simulink model "c221127_FCEV_SLMP_SQP"  (R2022b)
settings: Solver=FixedStepAuto  StartTime=0.0  StopTime=DrvCycLen  FixedStep=1  RelTol=1e-3
values from neighbouring files (symbols this model uses):
  AccThrshd = 1    [Config_c221112.m]    (also in Config_c221127.m; Config_c221218.m; Config_c230117.m; Config_c230321.m)
  AlphaRampFactor = 8    [Config_c221112.m]    (also in Config_c221127.m; Config_c221218.m; Config_c230117.m; Config_c230321.m)
  Bat_eff_chg_average = 0.969    [FCEV_original_data.mat]
  Bat_eff_dis_average = 0.9632    [FCEV_original_data.mat]
  Bat_end_of_life_percent = 20    [FCEV_original_data.mat]
  Bat_I_chg_max = -120    [FCEV_original_data.mat]
  Bat_I_dis_max = 200    [FCEV_original_data.mat]
  Bat_nom_Ic = 2.5    [FCEV_original_data.mat]
  Bat_nom_SOC = 0.35    [FCEV_original_data.mat]
  Bat_nom_temp_oC = 25    [FCEV_original_data.mat]
  Bat_num_pa = 9    [FCEV_original_data.mat]
  Bat_num_se = 97    [FCEV_original_data.mat]
  Bat_ori_C1_chg_F = [397.526659684 455.660832136 435.08783522 460.845064365 457.605812374 417.289828504 416.373906992 359.741413056 321.561704819 1109.14132554 1165.67733205 1135.97600211 ... (72 elements, 9x8)]    [FCEV_original_data.mat]
  Bat_ori_C1_dis_F = [187.121968588 287.083505726 346.448009002 395.529439835 387.517274826 389.973134196 432.856765051 486.92921923 512.158935268 425.990733989 614.68708868 771.472592368 ... (72 elements, 9x8)]    [FCEV_original_data.mat]
  Bat_ori_C2_chg_F = [8748.48589695 7773.35875681 9404.86567646 8934.73981058 8290.58671366 7592.78422269 7759.44623103 7396.59043829 6151.35152293 16187.7227039 11721.8480541 13157.8579836 ... (72 elements, 9x8)]    [FCEV_original_data.mat]
  Bat_ori_C2_dis_F = [2939.81325553 4590.73311898 5504.93546413 5887.5077374 6534.37836712 7765.46899768 10584.7751706 10372.0508438 9238.72693885 5207.86390693 7911.43744944 8879.62137571 ... (72 elements, 9x8)]    [FCEV_original_data.mat]
  Bat_ori_cap_max_Ah = 20.7    [Config_c221218.m]    (also in Config_c230117.m; Config_c230321.m; FCEV_original_data.mat)
  Bat_ori_dUdt4 = [-0.303773584906 -0.249056603774 -0.115094339623 -0.0396226415094 0.0396226415094 0.0641509433962 0.107547169811 0.111320754717 0.0415094339623 0.0547169811321 0.130188679245]    [FCEV_original_data.mat]
  Bat_ori_R0_chg_O = [0.0771669453735 0.0731809311402 0.0726556782939 0.0729965156794 0.0731758310684 0.0742031005051 0.0721266921026 0.0714211058078 0.0714186176143 0.0374124505155 0.0354566732504 0.0345430657188 ... (72 elements, 9x8)]    [FCEV_original_data.mat]
  Bat_ori_R0_dis_O = [0.0819458671157 0.0812429476608 0.0803749674507 0.0805513601722 0.0838629023857 0.0850797840015 0.0829875518672 0.0826388888889 0.0812514106148 0.0428124986417 0.0424658903711 0.0428572670451 ... (72 elements, 9x8)]    [FCEV_original_data.mat]
  Bat_ori_R1_chg_O = [0.114339870884 0.105392753268 0.104421193553 0.109821896183 0.114868279838 0.123333154908 0.129174812826 0.149917249373 0.174896487845 0.0420560161846 0.0390948352938 0.0370122837364 ... (72 elements, 9x8)]    [FCEV_original_data.mat]
  Bat_ori_R1_dis_O = [0.304806399643 0.213604089624 0.171463520004 0.151183840498 0.140630862434 0.128795299077 0.116857791733 0.112567113582 0.106368362501 0.0943235089866 0.0730697254134 0.0611414736086 ... (72 elements, 9x8)]    [FCEV_original_data.mat]
  Bat_ori_R2_chg_O = [0.134518959939 0.17565045702 0.161100627268 0.189032232545 0.205639040497 0.226170473035 0.223651875822 0.181765694192 0.212966950836 0.073628872144 0.0788540822416 0.0792414571734 ... (72 elements, 9x8)]    [FCEV_original_data.mat]
  Bat_ori_R2_dis_O = [0.354968099904 0.285293035102 0.286338708953 0.298763853987 0.248762838155 0.178586175471 0.129047399775 0.188406991173 0.174494800676 0.131839238891 0.123225430215 0.132069033134 ... (72 elements, 9x8)]    [FCEV_original_data.mat]
  Bat_ori_SOC2 = [0 0.001 0.002 0.003 0.004 0.005 0.006 0.007 0.008 0.009 0.01 0.011 ... (1001 elements, 1x1001)]    [FCEV_original_data.mat]
  Bat_ori_SOC4 = [-0.00598301069999 0.0920117618231 0.190864167279 0.289083557951 0.387343788287 0.485011843502 0.5850485992 0.678163031937 0.774810095565 0.876684636119 0.972739524626]    [FCEV_original_data.mat]
  Bat_ori_Uoc_chg_V = [2.4478 2.54923264342 2.6007 2.6383 2.66953057366 2.69636321708 2.7197 2.74042850391 2.75906114733 2.77619379074 2.792 2.80675907757 ... (1001 elements, 1x1001)]    [FCEV_original_data.mat]
  Bat_ori_Uoc_dis_V = [1.9998 2.03916768329 2.24724374236 2.39700902919 2.48767431602 2.5476 2.5882 2.6202 2.64771773167 2.6719 2.6933 2.71251566192 ... (1001 elements, 1x1001)]    [FCEV_original_data.mat]
  Bat_ori_Uoc_V = [2.2238 2.29420016335 2.42397187118 2.5176545146 2.57860244484 2.62198160854 2.65395 2.68031425195 2.7033894395 2.72404689537 2.74265 2.75963736975 ... (1001 elements, 1x1001)]    [FCEV_original_data.mat]
  Bat_power_max_kW = 50    [FCEV_original_data.mat]
  Bat_power_min_kW = 0    [FCEV_original_data.mat]
  Bat_single_capacity_nom_Ah = 2.3    [FCEV_original_data.mat]
  Bat_SOC_ini = 0.3    [Config_c22100601.m]    (also in Config_c22100701.m; FCEV_original_data.mat = 0.45)
  Bat_SOC_max = 0.9    [FCEV_original_data.mat]
  Bat_SOC_min = 0.3    [FCEV_original_data.mat]
  Bat_temp_amb_oC = 25    [FCEV_original_data.mat]
  Bat_temp_cool_oC = 25    [FCEV_original_data.mat]
  BattInitTemp = 25    [Config_c221127.m]    (also in Config_c221218.m; Config_c230117.m; Config_c230321.m)
  BattOnly = 0    [Config_c221218.m]    (also in Config_c230117.m = BattSocRightNow > BattSocLowerLimit; Config_c230321.m = double(BattSocRightNow > BattSocLowerLimit))
  BattSocInit = 0.9    [Config_c221112.m]    (also in Config_c221127.m = 0.3; Config_c221218.m = 0.3; Config_c230117.m = 0.8; Config_c230321.m = 0.8)
  BattSocLowerLimit = 0.25    [Config_c221112.m]    (also in Config_c221127.m = 0.3; Config_c221218.m = 0.3; Config_c230117.m = 0.3; Config_c230321.m = 0.3)
  BattSocRightNow = BattSocRightNow - SocDrop    [Config_c221218.m]    (also in Config_c230117.m; Config_c230321.m)
  BattSocUpperLimit = 0.9    [Config_c221112.m]    (also in Config_c221127.m = 0.8; Config_c221218.m = 0.8; Config_c230117.m = 0.8; Config_c230321.m = 0.8)
  CFWF = 0.5    [Config_c221127.m]    (also in Config_c221218.m; Config_c230117.m; Config_c230321.m)
  DCAC_eff = 0.95    [FCEV_original_data.mat]
  DCDC_ori_eff = [0.95 0.96 0.97 0.976 0.98 0.978 0.973 0.962]    [FCEV_original_data.mat]
  DCDC_ori_power_kW = [0 10 20 30 40 50 60 70]    [FCEV_original_data.mat]
  DeAccThrshd = -1    [Config_c221112.m]    (also in Config_c221127.m; Config_c221218.m; Config_c230117.m; Config_c230321.m)
  DeltaFcPwrRcm_down = 0.5    [Config_c221127.m]    (also in Config_c221218.m; Config_c230117.m; Config_c230321.m)
  DeltaFcPwrRcm_up = 2    [Config_c221127.m]    (also in Config_c221218.m = 3; Config_c230117.m = 4; Config_c230321.m = 4)
  DrvCycRange = sum(DrvCycVps(:,2))    [Config_c221112.m]    (also in Config_c221127.m; Config_c221218.m; Config_c230117.m; Config_c230321.m)
  FC_ori_eff = [0.1 0.33 0.492 0.533 0.559 0.596 0.591 0.562 0.508]    [FCEV_original_data.mat]
  FC_ori_fuel_rate_gps = [0 0.0505050505051 0.0846883468835 0.117260787992 0.149075730471 0.279642058166 0.423011844332 0.593119810202 0.820209973753]    [FCEV_original_data.mat]
  FC_ori_power_kW = [0 2 5 7.5 10 20 30 40 50]    [FCEV_original_data.mat]
  FC_power_max_kW = 50    [FCEV_original_data.mat]
  FC_power_min_kW = 0    [FCEV_original_data.mat]
  FcPwrDropCall = 6    [Config_c221127.m]    (also in Config_c221218.m; Config_c230117.m; Config_c230321.m)
  HydpriceRmb = 30    [Config_c221127.m]    (also in Config_c221218.m; Config_c230117.m; Config_c230321.m)
  m = Time_sample    [Config_c22100601.m]    (also in Config_c22100701.m)
  MC_eff_brk_average = 0.810578512397    [FCEV_original_data.mat]
  MC_eff_dri_average = 0.810578512397    [FCEV_original_data.mat]
  MC_inertia = 0.06    [FCEV_original_data.mat]
  MC_ori_eff = [0.7 0.78 0.85 0.86 0.81 0.82 0.79 0.78 0.78 0.78 0.78 0.7 ... (231 elements, 11x21)]    [FCEV_original_data.mat]
  MC_ori_power_brk_req_kW = [0 -28.3912930389 -56.7825860779 -85.1738791168 -113.565172156 -141.956465195 -170.347758234 -198.739051273 -227.130344311 -255.52163735 -283.912930389 0 ... (121 elements, 11x11)]    [FCEV_original_data.mat]
  MC_ori_power_dri_req_kW = [0 0 0 0 0 0 0 0 0 0 0 0 ... (121 elements, 11x11)]    [FCEV_original_data.mat]
  MC_ori_spd_rpm = [0 1000 2000 3000 4000 5000 6000 7000 8000 9000 10000]    [FCEV_original_data.mat]
  MC_ori_trq_brk_max_Nm = [-271.1368 -271.1368 -271.1368 -237.5159 -178.1369 -142.4824 -118.7579 -101.8119 -89.0685 -79.172 -71.1734]    [FCEV_original_data.mat]
  MC_ori_trq_brk_Nm = [-271.136848522 -244.02316367 -216.909478817 -189.795793965 -162.682109113 -135.568424261 -108.454739409 -81.3410545565 -54.2273697044 -27.1136848522 0]    [FCEV_original_data.mat]
  MC_ori_trq_dri_max_Nm = [271.1368 271.1368 271.1368 237.5159 178.1369 142.4824 118.7579 101.8119 89.0685 79.172 71.1734]    [FCEV_original_data.mat]
  MC_ori_trq_dri_Nm = [0 27.1136848522 54.2273697044 81.3410545565 108.454739409 135.568424261 162.682109113 189.795793965 216.909478817 244.02316367 271.136848522]    [FCEV_original_data.mat]
  MC_ori_trq_Nm = [-271.136848522 -244.02316367 -216.909478817 -189.795793965 -162.682109113 -135.568424261 -108.454739409 -81.3410545565 -54.2273697044 -27.1136848522 0 27.1136848522 ... (21 elements, 1x21)]    [FCEV_original_data.mat]
  MC_power_max_kW = 75    [FCEV_original_data.mat]
  MC_spd_max_rpm = 10000    [FCEV_original_data.mat]
  MC_spd_min_rpm = 0    [FCEV_original_data.mat]
  MC_spd_scale = 1    [FCEV_original_data.mat]
  MC_trq_scale = 1    [FCEV_original_data.mat]
  MC_U_min_V = 120    [FCEV_original_data.mat]
  no_FcPwrSlowDrop = 1    [Config_c230321.m]
  Placeholder = 0    [Config_c221127.m]    (also in Config_c221218.m; Config_c230117.m; Config_c230321.m)
  PredLen = 5    [Config_c221112.m]    (also in Config_c221127.m; Config_c221218.m; Config_c230117.m; Config_c230321.m)
  Road_u = 0.75    [FCEV_original_data.mat]
  SC_np = 1    [Config_c230321.m]
  SC_ns = 100    [Config_c230321.m]
  SC_rc = 1000    [Config_c230321.m]
  SLMP_LearningRate = 0.05    [Config_c221112.m]    (also in Config_c221127.m; Config_c221218.m; Config_c230117.m; Config_c230321.m)
  tDegTable = [zeros(1,3),linspace(0,0.13,47)]    [Config_c221127.m]    (also in Config_c221218.m; Config_c230117.m; Config_c230321.m)
  usd2rmb = 7.116    [Config_c22100601.m]    (also in Config_c22100701.m; Config_c221106.m = 6; Config_c221112.m = 6; Config_c221127.m = 6)
  Veh_air_density_kgpm2 = 1.2    [FCEV_original_data.mat]
  Veh_brk_front = [1 0.6 0.608 0.61 0.618 0.624 0.636 0.645 0.655]    [FCEV_original_data.mat]
  Veh_brk_z = [0.1 0.2 0.3 0.4 0.5 0.6 0.7 0.8 0.9]    [FCEV_original_data.mat]
  Veh_brk_z_max = 0.7    [FCEV_original_data.mat]
  Veh_brk_z_min = 0.1    [FCEV_original_data.mat]
  Veh_coeff_drag = 0.312    [FCEV_original_data.mat]
  Veh_coeff_roll = 0.00863    [FCEV_original_data.mat]
  Veh_final_drive_inertia = 0.1105    [FCEV_original_data.mat]
  Veh_final_drive_ratio = 3.47    [FCEV_original_data.mat]
  Veh_frontal_area_m2 = 2.06    [FCEV_original_data.mat]
  Veh_gravity_acc_ms2 = 9.81    [FCEV_original_data.mat]
  Veh_mass_cargo_kg = 113    [FCEV_original_data.mat]
  Veh_mass_curb_kg = 1157    [FCEV_original_data.mat]
  Veh_mech_eff = 0.9    [FCEV_original_data.mat]
  Veh_rotary_mass_conversion_factor = 1.05    [FCEV_original_data.mat]
  Veh_size_cg_height_m = 0.53    [FCEV_original_data.mat]
  Veh_wheel_inertia = 3.1039    [FCEV_original_data.mat]
  Veh_wheel_radius_m = 0.313    [FCEV_original_data.mat]
  Veh_wt_frac_front = 0.5    [FCEV_original_data.mat]
  VstdThrshd = 2    [Config_c221112.m]    (also in Config_c221127.m; Config_c221218.m; Config_c230117.m; Config_c230321.m)
undefined symbols (not defined in the file or in its folder): Bat_ori_temp, SC_iv, SC_nm, SC_SocTable
libraries: autolibshared x2
(part 3 of 8)

== system c221127_FCEV_SLMP_SQP/VehModel_Current/车轮模型 ==
  "tractive force, brake force and speed req'd of tire/road interface 需求驱动力N 目标车速m/s 需求制动力N" : Inport
  "drive torque (Nm) brake torque (Nm) speed (rad/s) available from drivetrain into axle " : Inport  Port=2
  - : Gain  Gain=Veh_wheel_radius_m
  Add : Sum
  Add1 : Sum
  Add2 : Sum  Inputs=-+
  Add3 : Sum  Inputs=-+
  Constant : Constant  Value=0
  Demux : Demux  Outputs=3
  Demux1 : Demux  Outputs=3
  Gain1 : Gain  Gain=Veh_wheel_radius_m
  Gain2 : Gain  Gain=1/Veh_wheel_radius_m
  Gain3 : Gain  Gain=1/Veh_wheel_radius_m
  Gain4 : Gain  Gain=Veh_wheel_radius_m
  Interia torque : Subsystem
  Interia torque1 : Subsystem
  Mux : Mux  Inputs=3
  Mux3 : Mux  Inputs=3
  Regenerative energy compute : Subsystem
  Saturation : Saturate  UpperLimit=inf  LowerLimit=0
  Saturation1 : Saturate  UpperLimit=0  LowerLimit=-inf
  Scope : Scope
  Switch1 : Switch  Criteria=u2 > Threshold  Threshold=15  SaturateOnIntegerOverflow=off  InputSameDT=off
  Tire slip model : Subsystem
  Tire slip model1 : Subsystem
  axle input speed (rad/s) : Gain  Gain=1/Veh_wheel_radius_m
  drive torque (Nm) speed (rad/s) brake torque (Nm) req'd from drivetrain into axle : Outport  InitialOutput=0
  tractive force (N) brake force (N) linear speed achievable (m/s) : Outport  Port=2  InitialOutput=0
  wires:
  Demux/1 -> Gain1/1
  "tractive force, brake force and speed req'd of tire/road interface 需求驱动力N 目标车速m/s 需求制动力N"/1 -> Demux/1
  "drive torque (Nm) brake torque (Nm) speed (rad/s) available from drivetrain into axle "/1 -> Demux1/1
  Demux1/1 -> Add2/2
  Mux/1 -> drive torque (Nm) speed (rad/s) brake torque (Nm) req'd from drivetrain into axle/1
  Gain1/1 -> Add/2
  Add/1 -> Mux/1
  Add2/1 -> Gain2/1
  Gain2/1 -> Tire slip model/1(In1)
  Mux3/1 -> Scope/1, tractive force (N) brake force (N) linear speed achievable (m/s)/1
  Demux/2 -> axle input speed (rad/s)/1, Interia torque/1(车轮线速度 m/s), Interia torque1/1(车轮线速度 m/s)
  Interia torque/1(inertia torque (Nm)) -> Add2/1, Add/1
  Demux/3 -> Gain4/1
  Gain4/1 -> Add1/1
  Interia torque1/1(inertia torque (Nm)) -> Add3/1, Add1/2
  axle input speed (rad/s)/1 -> Switch1/2, Mux/2
  Switch1/1 -> Mux/3
  Constant/1 -> Switch1/3
  Add1/1 -> Switch1/1
  Saturation/1 -> Mux3/1
  Tire slip model/1(dri_force available in front wheel n) -> Saturation/1
  Tire slip model1/1(brk_force available in front wheel n) -> Saturation1/1
  Saturation1/1 -> Regenerative energy compute/1(motor brk force), Mux3/2
  Gain3/1 -> Tire slip model1/1(In1)
  Demux1/2 -> Add3/2
  Add3/1 -> Gain3/1
  Demux1/3 -> -/1
  -/1 -> Regenerative energy compute/3(spd2), Regenerative energy compute/2(spd), Mux3/3

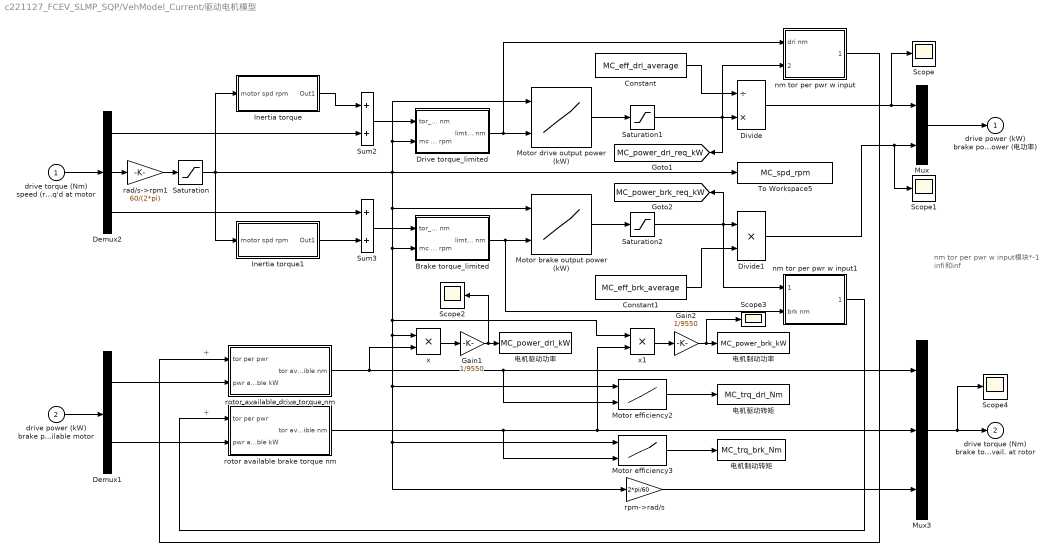
== system c221127_FCEV_SLMP_SQP/VehModel_Current/驱动电机模型 ==
  note: +
  note: +
  note: nm tor per pwr w input模块*-1
      | infi和inf
  drive torque (Nm) speed (rad/s) brake torque (Nm) req'd at motor : Inport
  drive power (kW) brake power (kW) input available motor : Inport  Port=2
  Brake torque_limited : Subsystem
  Constant : Constant  Value=MC_eff_dri_average
  Constant1 : Constant  Value=MC_eff_brk_average
  Demux1 : Demux  Outputs=2
  Demux2 : Demux  Outputs=3
  Divide : Product  Inputs=/*
  Divide1 : Product  Inputs=**
  Drive torque_limited : Subsystem
  Gain1 : Gain  Gain=1/9550
  Gain2 : Gain  Gain=1/9550
  Inertia torque : Subsystem
  Inertia torque1 : Subsystem
  Motor brake output power (kW) : Lookup2D  RowIndex=MC_ori_spd_rpm*MC_spd_scale  ColumnIndex=MC_ori_trq_brk_Nm*MC_trq_scale  Table=MC_ori_power_brk_req_kW*MC_spd_scale*MC_trq_scale
  Motor drive output power (kW) : Lookup2D  RowIndex=MC_ori_spd_rpm*MC_spd_scale  ColumnIndex=MC_ori_trq_dri_Nm*MC_trq_scale  Table=MC_ori_power_dri_req_kW*MC_spd_scale*MC_trq_scale
  Motor efficiency2 : Lookup2D  RowIndex=MC_ori_spd_rpm*MC_spd_scale  ColumnIndex=MC_ori_trq_Nm*MC_trq_scale  Table=MC_ori_eff*MC_spd_scale*MC_trq_scale
  Motor efficiency3 : Lookup2D  RowIndex=MC_ori_spd_rpm*MC_spd_scale  ColumnIndex=MC_ori_trq_Nm*MC_trq_scale  Table=MC_ori_eff*MC_spd_scale*MC_trq_scale
  Mux : Mux  Inputs=2
  Mux3 : Mux  Inputs=3
  Saturation : Saturate  UpperLimit=MC_spd_max_rpm  LowerLimit=MC_spd_min_rpm
  Saturation1 : Saturate  UpperLimit=MC_power_max_kW  LowerLimit=0  LinearizeAsGain=off
  Saturation2 : Saturate  UpperLimit=0  LowerLimit=-MC_power_max_kW
  Scope{,1..4} (5 alike) : Scope
  Sum2 : Sum  InputSameDT=on  SaturateOnIntegerOverflow=on  OutDataTypeStr=Inherit: Same as first input
  Sum3 : Sum  InputSameDT=on  SaturateOnIntegerOverflow=on  OutDataTypeStr=Inherit: Same as first input
  To Workspace5 : ToWorkspace  VariableName=MC_spd_rpm  SampleTime=-1
  nm tor per pwr w input : Subsystem
  nm tor per pwr w input1 : Subsystem
  rad/s->rpm1 : Gain  Gain=60/(2*pi)
  rotor available brake torque nm : Subsystem
  rotor available drive torque nm : Subsystem
  rpm->rad/s : Gain  Gain=2*pi/60
  x : Product  Inputs=**
  x1 : Product  Inputs=**
  电机制动功率 : ToWorkspace  VariableName=MC_power_brk_kW  SampleTime=-1
  电机制动转矩 : ToWorkspace  VariableName=MC_trq_brk_Nm  SampleTime=-1
  电机驱动功率 : ToWorkspace  VariableName=MC_power_dri_kW  SampleTime=-1
  电机驱动转矩 : ToWorkspace  VariableName=MC_trq_dri_Nm  SampleTime=-1
  drive power (kW) brake power (kW) req'd motor input power (电功率) : Outport  InitialOutput=0
  drive torque (Nm) brake torque (Nm) speed avail (rad/s) avail. at rotor : Outport  Port=2  InitialOutput=0
  tag scope: MC_power_brk_req_kW=global, MC_power_dri_req_kW=global
  wires:
  drive torque (Nm) speed (rad/s) brake torque (Nm) req'd at motor/1 -> Demux2/1
  rad/s->rpm1/1 -> Saturation/1
  Demux2/2 -> rad/s->rpm1/1
  Demux2/1 -> Sum2/2
  Inertia torque/1(Out1) -> Sum2/1
  Sum2/1 -> Drive torque_limited/1(tor_req nm)
  Drive torque_limited/1(limted mc torque nm) -> Motor drive output power (kW)/2, nm tor per pwr w input/1(dri nm)
  Motor drive output power (kW)/1 -> Saturation1/1
  Constant/1 -> Divide/1
  Divide/1 -> Scope/1, Mux/1
  Mux/1 -> drive power (kW) brake power (kW) req'd motor input power (电功率)/1
  Demux2/3 -> Sum3/1
  Inertia torque1/1(Out1) -> Sum3/2
  Sum3/1 -> Brake torque_limited/1(tor_req nm)
  Motor brake output power (kW)/1 -> Saturation2/1
  Saturation2/1 -> [MC_power_brk_req_kW], nm tor per pwr w input1/1(pwr brk kW), Divide1/1
  Constant1/1 -> Divide1/2
  Divide1/1 -> Scope1/1, Mux/2
  drive power (kW) brake power (kW) input available motor/1 -> Demux1/1
  Saturation1/1 -> nm tor per pwr w input/2(pwr dri kW), [MC_power_dri_req_kW], Divide/2
  Demux1/1 -> rotor available drive torque nm/2(pwr available kW)
  nm tor per pwr w input/1(tor per pwr) -> rotor available drive torque nm/1(tor per pwr)
  Demux1/2 -> rotor available brake torque nm/2(pwr available kW)
  nm tor per pwr w input1/1(tor per pwr) -> rotor available brake torque nm/1(tor per pwr)
  rotor available brake torque nm/1(tor avaible nm) -> Motor efficiency3/2, x1/2, Mux3/2
  rotor available drive torque nm/1(tor avaible nm) -> Motor efficiency2/2, Mux3/1, x/2
  rpm->rad/s/1 -> Mux3/3
  Motor efficiency3/1 -> 电机制动转矩/1
  Motor efficiency2/1 -> 电机驱动转矩/1
  Brake torque_limited/1(limted mc torque nm) -> nm tor per pwr w input1/2(brk nm), Motor brake output power (kW)/2
  Gain1/1 -> Scope2/1, 电机驱动功率/1
  x/1 -> Gain1/1
  Gain2/1 -> Scope3/1, 电机制动功率/1
  x1/1 -> Gain2/1
  Saturation/1 -> Inertia torque1/1(motor spd rpm), x1/1, x/1, Motor efficiency2/1, Motor efficiency3/1, rpm->rad/s/1, Brake torque_limited/2(mc spd rpm), Motor brake output power (kW)/1, To Workspace5/1, Motor drive output power (kW)/1, Drive torque_limited/2(mc spd rpm), Inertia torque/1(motor spd rpm)
  Mux3/1 -> Scope4/1, drive torque (Nm) brake torque (Nm) speed avail (rad/s) avail. at rotor/1

== system c221127_FCEV_SLMP_SQP/Subsystem2/Capacity Degradation Model (Cell)1/计算实际寿命 ==
  note: 参考文献：A control-oriented cycle-life model for hybrid electric vehicle lithiumion batteries
  note: Beta
  note: Alpha
  温度 : Inport
  倍率 : Inport  Port=2
  SOC : Inport  Port=3
  -31700+163.3*Ic : Sum  InputSameDT=on  SaturateOnIntegerOverflow=on  OutDataTypeStr=Inherit: Same as first input
  Alpha*SOC+Beta1 : Sum  InputSameDT=on  SaturateOnIntegerOverflow=on  OutDataTypeStr=Inherit: Same as first input
  Alpha3 : Constant  Value=2896.6
  Alpha4 : Constant  Value=2649.5
  Beta3 : Constant  Value=7411.2
  Beta4 : Constant  Value=6022.2
  Constant : Constant  Value=-31500
  Constant1 : Constant  Value=152.5
  Constant2 : Constant  Value=273.15
  Fcn2 : Fcn  Expr=u^(1/0.57)
  Math Function : Math  Operator=reciprocal  SignedPower=on
  Math Function1 : Math  Operator=reciprocal  SignedPower=on
  Math Function2 : Math  SignedPower=on
  R : Constant  Value=8.314
  R*T : Product  InputSameDT=on  RndMeth=Zero  SaturateOnIntegerOverflow=on  OutDataTypeStr=Inherit: Same as first input
  Switch3 : Switch  Criteria=u2 > Threshold  Threshold=0.45
  Switch4 : Switch  Criteria=u2 > Threshold  Threshold=0.45
  severity factor function : Product  InputSameDT=on  RndMeth=Zero  SaturateOnIntegerOverflow=on  OutDataTypeStr=Inherit: Same as first input
  x : Product  InputSameDT=on  RndMeth=Zero  SaturateOnIntegerOverflow=on  OutDataTypeStr=Inherit: Same as first input
  x1 : Product  InputSameDT=on  RndMeth=Zero  SaturateOnIntegerOverflow=on  OutDataTypeStr=Inherit: Same as first input
  x2 : Product  InputSameDT=on  RndMeth=Zero  SaturateOnIntegerOverflow=on  OutDataTypeStr=Inherit: Same as first input
  ×1 : Product  InputSameDT=on  RndMeth=Zero  SaturateOnIntegerOverflow=on  OutDataTypeStr=Inherit: Same as first input
  ℃->开氏温度(绝对温度) : Sum  InputSameDT=on  SaturateOnIntegerOverflow=on  OutDataTypeStr=Inherit: Same as first input
  电池标准状态寿命 : ToWorkspace  VariableName=Bat_life_nom  SampleTime=-1
  电池终止寿命(%) : Constant  Value=Bat_end_of_life_percent
  Bat_life_nom : Outport
  wires:
  R/1 -> R*T/1
  ℃->开氏温度(绝对温度)/1 -> R*T/2
  Constant/1 -> -31700+163.3*Ic/1
  x/1 -> -31700+163.3*Ic/2
  Constant1/1 -> x/1
  -31700+163.3*Ic/1 -> x1/1
  R*T/1 -> Math Function/1
  Math Function/1 -> x1/2
  x1/1 -> Math Function2/1
  温度/1 -> ℃->开氏温度(绝对温度)/1
  Constant2/1 -> ℃->开氏温度(绝对温度)/2
  倍率/1 -> x/2
  Math Function2/1 -> severity factor function/1
  Alpha*SOC+Beta1/1 -> severity factor function/2
  severity factor function/1 -> Math Function1/1
  电池终止寿命(%)/1 -> x2/1
  Math Function1/1 -> x2/2
  x2/1 -> Fcn2/1
  Fcn2/1 -> Bat_life_nom/1, 电池标准状态寿命/1
  SOC/1 -> Switch4/2, ×1/1, Switch3/2
  Alpha4/1 -> Switch3/1
  Alpha3/1 -> Switch3/3
  Beta4/1 -> Switch4/1
  Beta3/1 -> Switch4/3
  Switch3/1 -> ×1/2
  Switch4/1 -> Alpha*SOC+Beta1/2
  ×1/1 -> Alpha*SOC+Beta1/1

== system c221127_FCEV_SLMP_SQP/Subsystem2/Capacity Degradation Model (Cell)1/计算电池寿命(标准条件下) ==
  note: 参考文献：A control-oriented cycle-life model for hybrid electric vehicle lithiumion batteries
  note: Beta
  note: Alpha
  标准温度 : Inport
  标准倍率 : Inport  Port=2
  标准SOC : Inport  Port=3
  -31500+152.5*Ic : Sum  InputSameDT=on  SaturateOnIntegerOverflow=on  OutDataTypeStr=Inherit: Same as first input
  Alpha*SOC+Beta : Sum  InputSameDT=on  SaturateOnIntegerOverflow=on  OutDataTypeStr=Inherit: Same as first input
  Alpha3 : Constant  Value=2896.6
  Alpha4 : Constant  Value=2649.5
  Beta3 : Constant  Value=7411.2
  Beta4 : Constant  Value=6022.2
  Constant : Constant  Value=-31500
  Constant1 : Constant  Value=152.5
  Constant2 : Constant  Value=273.15
  Fcn2 : Fcn  Expr=u^(1/0.57)
  Math Function : Math  Operator=reciprocal  SignedPower=on
  Math Function1 : Math  Operator=reciprocal  SignedPower=on
  Math Function2 : Math  SignedPower=on
  R : Constant  Value=8.314
  R*T : Product  InputSameDT=on  RndMeth=Zero  SaturateOnIntegerOverflow=on  OutDataTypeStr=Inherit: Same as first input
  Switch3 : Switch  Criteria=u2 > Threshold  Threshold=0.45
  Switch4 : Switch  Criteria=u2 > Threshold  Threshold=0.45
  severity factor function : Product  InputSameDT=on  RndMeth=Zero  SaturateOnIntegerOverflow=on  OutDataTypeStr=Inherit: Same as first input
  x : Product  InputSameDT=on  RndMeth=Zero  SaturateOnIntegerOverflow=on  OutDataTypeStr=Inherit: Same as first input
  x1 : Product  InputSameDT=on  RndMeth=Zero  SaturateOnIntegerOverflow=on  OutDataTypeStr=Inherit: Same as first input
  x2 : Product  InputSameDT=on  RndMeth=Zero  SaturateOnIntegerOverflow=on  OutDataTypeStr=Inherit: Same as first input
  ×1 : Product  InputSameDT=on  RndMeth=Zero  SaturateOnIntegerOverflow=on  OutDataTypeStr=Inherit: Same as first input
  ℃->开氏温度(绝对温度) : Sum  InputSameDT=on  SaturateOnIntegerOverflow=on  OutDataTypeStr=Inherit: Same as first input
  电池实际状态寿命 : ToWorkspace  VariableName=Bat_life_act  SampleTime=-1
  电池终止寿命(%) : Constant  Value=Bat_end_of_life_percent
  Bat_life_act : Outport
  wires:
  R/1 -> R*T/1
  ℃->开氏温度(绝对温度)/1 -> R*T/2
  Constant/1 -> -31500+152.5*Ic/1
  x/1 -> -31500+152.5*Ic/2
  Constant1/1 -> x/1
  -31500+152.5*Ic/1 -> x1/1
  R*T/1 -> Math Function/1
  Math Function/1 -> x1/2
  x1/1 -> Math Function2/1
  标准温度/1 -> ℃->开氏温度(绝对温度)/1
  Constant2/1 -> ℃->开氏温度(绝对温度)/2
  标准倍率/1 -> x/2
  Math Function2/1 -> severity factor function/1
  Alpha*SOC+Beta/1 -> severity factor function/2
  severity factor function/1 -> Math Function1/1
  电池终止寿命(%)/1 -> x2/1
  Math Function1/1 -> x2/2
  x2/1 -> Fcn2/1
  Fcn2/1 -> Bat_life_act/1, 电池实际状态寿命/1
  标准SOC/1 -> Switch4/2, ×1/1, Switch3/2
  Alpha4/1 -> Switch3/1
  Alpha3/1 -> Switch3/3
  Beta4/1 -> Switch4/1
  Beta3/1 -> Switch4/3
  Switch3/1 -> ×1/2
  Switch4/1 -> Alpha*SOC+Beta/2
  ×1/1 -> Alpha*SOC+Beta/1

== system c221127_FCEV_SLMP_SQP/Subsystem2/Electrical Model1/Current calculation ==
  note: #:电池单体水平
  note: R0chg
  note: R0dis
  Voc : Inport
  Rint : Inport  Port=2
  limited output power (W) : Inport  Port=3
  Constant : Constant  Value=Bat_I_chg_max
  Constant1 : Constant  Value=Bat_I_dis_max
  Constant2 : Constant  Value=0
  Demux : Demux  Outputs=2
  Ibty=(Voc-(Voc^2-4RPbty)^.5) ----------------------------- (2*R) : Fcn  Expr=(u[2]-(u[2]^2-4*u[1]*u[3])^.5)/(2*u[3])
  Ibty=(Voc-(Voc^2-4RPbty)^.5) ----------------------------- (2*R)1 : Fcn  Expr=(u[2]-(u[2]^2-4*u[1]*u[3])^.5)/(2*u[3])
  MinMax : MinMax  Inputs=2
  MinMax1 : MinMax  Function=max  Inputs=2
  Mux : Mux  Inputs=2
  Mux1 : Mux  Inputs=3
  Mux2 : Mux  Inputs=3
  Pbat->Pcell : Gain  Gain=1/(Bat_num_pa*Bat_num_se)  SaturateOnIntegerOverflow=on  OutDataTypeStr=Inherit: Same as input  ParamDataTypeStr=Inherit: Same as input
  Scope : Scope
  Scope1 : Scope
  Switch : Switch  Criteria=u2 > Threshold
  Switch1 : Switch  Criteria=u2 > Threshold  SaturateOnIntegerOverflow=off  InputSameDT=off
  Switch2 : Switch  Criteria=u2 > Threshold
  I_dis (A) I_chg (A) Cell : Outport  InitialOutput=0
  I (A) Cell : Outport  Port=2  InitialOutput=0
  wires:
  Rint/1 -> Demux/1
  limited output power (W)/1 -> Pbat->Pcell/1
  Pbat->Pcell/1 -> Switch/1, Switch/2, Switch2/3, Switch2/2, Switch1/2
  Mux1/1 -> Ibty=(Voc-(Voc^2-4RPbty)^.5) ----------------------------- (2*R)/1
  Demux/1 -> Mux1/3
  Voc/1 -> Mux1/2, Mux2/2
  Demux/2 -> Mux2/3
  Mux2/1 -> Ibty=(Voc-(Voc^2-4RPbty)^.5) ----------------------------- (2*R)1/1
  Ibty=(Voc-(Voc^2-4RPbty)^.5) ----------------------------- (2*R)/1 -> MinMax/2
  Constant1/1 -> MinMax/1
  Ibty=(Voc-(Voc^2-4RPbty)^.5) ----------------------------- (2*R)1/1 -> MinMax1/1
  Constant/1 -> MinMax1/2
  MinMax/1 -> Switch1/1, Mux/1
  MinMax1/1 -> Mux/2, Switch1/3
  Mux/1 -> Scope/1, I_dis (A) I_chg (A) Cell/1
  Switch1/1 -> Scope1/1, I (A) Cell/1
  Switch/1 -> Mux1/1
  Switch2/1 -> Mux2/1
  Constant2/1 -> Switch/3, Switch2/1

== system c221127_FCEV_SLMP_SQP/Subsystem2/Electrical Model1/Entropic Heat ==
  note: 用于计算可逆热
  T : Inport
  SOC : Inport  Port=2
  Constant : Constant  Value=273
  Ent heat : Product  RndMeth=Zero
  Scope : Scope
  Sum2 : Sum  Inputs=|++
  dudT : Lookup  InputValues=Bat_ori_SOC4  Table=Bat_ori_dUdt4  SaturateOnIntegerOverflow=off
  mV->V : Gain  Gain=1/1000
  HG_ent : Outport
  wires:
  Sum2/1 -> Ent heat/2
  Constant/1 -> Sum2/2
  T/1 -> Sum2/1
  dudT/1 -> Ent heat/1
  Ent heat/1 -> mV->V/1
  SOC/1 -> dudT/1
  mV->V/1 -> Scope/1, HG_ent/1

== system c221127_FCEV_SLMP_SQP/Subsystem2/Electrical Model1/Limited power (Battery pack level) ==
  SOC : Inport
  Pbty : Inport  Port=2
  " " : RelationalOperator  Operator=>  OutDataTypeStr=boolean  InputSameDT=off
  " 1" : RelationalOperator  Operator=<  OutDataTypeStr=boolean  InputSameDT=off
  " 3" : Constant  Value=0.95
  Add : Sum
  Constant : Constant  Value=eps
  Constant1 : Constant  Value=eps
  Constant{2..5} (4 alike) : Constant  Value=0
  Logical Operator : Logic  Operator=OR  AllPortsSameDT=off  OutDataTypeStr=boolean
  Logical Operator1 : Logic  AllPortsSameDT=off  OutDataTypeStr=boolean
  Memory1 : Memory  InitialCondition=Bat_SOC_ini  InheritSampleTime=on
  Relational Operator : RelationalOperator  Operator=>  OutDataTypeStr=boolean  InputSameDT=off
  Relational Operator1 : RelationalOperator  OutDataTypeStr=boolean  InputSameDT=off
  Scope : Scope
  Scope1 : Scope  NumInputPorts=2
  Scope2 : Scope  NumInputPorts=2
  Scope3 : Scope
  Switch{,1..3} (4 alike) : Switch  Criteria=u2 > Threshold  Threshold=eps  SaturateOnIntegerOverflow=off  InputSameDT=off
  "Pbty, limited W" : Outport  InitialOutput=0
  wires:
  Memory1/1 -> Relational Operator/1, Relational Operator1/1, Scope3/1
  Constant/1 -> Relational Operator/2
  Relational Operator/1 -> Logical Operator/1
  Switch3/1 -> Scope2/2, " 1"/1, Switch1/3
  Constant1/1 -> " "/2
  " "/1 -> Logical Operator/2
  Logical Operator/1 -> Switch/2
  Constant2/1 -> Switch/3
  " 3"/1 -> Relational Operator1/2
  Relational Operator1/1 -> Logical Operator1/1
  Logical Operator1/1 -> Switch1/2
  Constant3/1 -> Switch1/1
  Constant4/1 -> " 1"/2
  " 1"/1 -> Logical Operator1/2
  Switch2/1 -> Scope2/1, " "/1, Switch/1
  Add/1 -> Scope/1, "Pbty, limited W"/1
  Switch/1 -> Scope1/1, Add/1
  Switch1/1 -> Add/2, Scope1/2
  Pbty/1 -> Switch2/1, Switch3/3, Switch3/2, Switch2/2
  Constant5/1 -> Switch3/1, Switch2/3
  SOC/1 -> Memory1/1

== system c221127_FCEV_SLMP_SQP/Subsystem2/Electrical Model1/Max power in W (Battery pack level) ==
  Constant3 : Constant  Value=Bat_I_dis_max
  Constant4 : Constant  Value=Bat_I_chg_max
  Max power in W (Battery pack level)1 : Subsystem
  Mux1 : Mux  Inputs=3
  Mux2 : Mux  Inputs=3
  Product : Product  InputSameDT=on  RndMeth=Zero  SaturateOnIntegerOverflow=on  OutDataTypeStr=Inherit: Same as first input
  Product1 : Product  InputSameDT=on  RndMeth=Zero  SaturateOnIntegerOverflow=on  OutDataTypeStr=Inherit: Same as first input
  R0,cell->R0,bat : Gain  Gain=Bat_num_se/Bat_num_pa  SaturateOnIntegerOverflow=on  OutDataTypeStr=Inherit: Same as input  ParamDataTypeStr=Inherit: Same as input
  R0,cell->R0,bat1 : Gain  Gain=Bat_num_se/Bat_num_pa  SaturateOnIntegerOverflow=on  OutDataTypeStr=Inherit: Same as input  ParamDataTypeStr=Inherit: Same as input
  fun : Fcn  Expr=u[2]-u[1]*u[3]
  fun1 : Fcn  Expr=u[2]-u[1]*u[3]
  max ess discharge pwr : Outport  InitialOutput=0
  max ess charge pwr : Outport  Port=2  InitialOutput=0
  wires:
  [Bat_R0_dis_O] -> R0,cell->R0,bat/1
  [Bat_R0_chg_O] -> R0,cell->R0,bat1/1
  Constant4/1 -> Product1/1, Mux2/1
  Constant3/1 -> Product/1, Mux1/1
  R0,cell->R0,bat/1 -> Mux1/3
  [Bat_Uoc_V] -> Mux2/2, Mux1/2
  Mux1/1 -> fun/1
  R0,cell->R0,bat1/1 -> Mux2/3
  Mux2/1 -> fun1/1
  fun/1 -> Product/2
  Product/1 -> max ess discharge pwr/1
  fun1/1 -> Product1/2
  Product1/1 -> max ess charge pwr/1

== system c221127_FCEV_SLMP_SQP/Subsystem2/Electrical Model1/Parameter Lookup2 ==
  note: #Cell Level
  SOC : Inport
  T : Inport  Port=2
  P : Inport  Port=3
  Gain{1..5} (5 alike) : Gain
  Lookup C1 : Subsystem
  Lookup C2 : Subsystem
  Lookup R1 : Subsystem
  Lookup R2 : Subsystem
  Lookup Rs : Subsystem
  Lookup Uoc : Subsystem
  Uoc : Outport
  R1 : Outport  Port=2
  C1 : Outport  Port=3
  R2 : Outport  Port=4
  C2 : Outport  Port=5
  R0 : Outport  Port=6
  wires:
  [BattSoc] -> Lookup Rs/1(SOC), Lookup R1/1(SOC), Lookup C1/1(SOC), Lookup Uoc/1(SOC), Lookup C2/1(SOC), Lookup R2/1(SOC1)
  [BattTemp] -> Lookup Rs/2(T), Lookup R1/2(T), Lookup C1/2(T), Lookup C2/2(T), Lookup R2/2(T)
  [BattPwr] -> Lookup R1/3(P), Lookup C1/3(P), Lookup C2/3(P), Lookup Uoc/2(P), Lookup R2/3(P)
  Gain3/1 -> C1/1
  Lookup C2/1(C2) -> Gain4/1
  Gain4/1 -> C2/1
  Gain2/1 -> R2/1
  Lookup R2/1(R2) -> Gain2/1
  Gain1/1 -> R1/1
  Lookup R1/1(R1) -> Gain1/1
  Lookup C1/1(C1) -> Gain3/1
  Lookup Uoc/1(Uoc) -> Gain5/1
  Gain5/1 -> Uoc/1
  Lookup Rs/1(R0) -> R0/1
  SOC/1 -> [BattSoc]
  T/1 -> [BattTemp]
  P/1 -> [BattPwr]

== system c221127_FCEV_SLMP_SQP/Subsystem2/Electrical Model1/SOC Calculation ==
  note: 充电
  note: 放电
  note: #:电池组水平
  I_dis (A) I_chg (A) : Inport
  (sec->hrs) : Gain  Gain=1/3600  SaturateOnIntegerOverflow=on  OutDataTypeStr=Inherit: Same as input  ParamDataTypeStr=Inherit: Same as input
  0 <= SOC <= 1 : Saturate  UpperLimit=1  LowerLimit=eps
  Add5 : Sum  Inputs=-+
  Add6 : Sum  Inputs=-+
  Bat SOC0 : Constant  Value=BattSocInit
  Bat chg eff : Constant  Value=Bat_eff_chg_average
  Bat dis eff : Constant  Value=Bat_eff_dis_average
  CD/CS mode judgement : Subsystem
  Demux : Demux  Outputs=2
  Divide1 : Product  Inputs=*/
  Divide3 : Product  Inputs=**
  Divide4 : Product  Inputs=*/
  Icell->Ibat : Gain  Gain=Bat_num_pa  SaturateOnIntegerOverflow=on  OutDataTypeStr=Inherit: Same as input  ParamDataTypeStr=Inherit: Same as input
  Icell->Ibat1 : Gain  Gain=Bat_num_pa  SaturateOnIntegerOverflow=on  OutDataTypeStr=Inherit: Same as input  ParamDataTypeStr=Inherit: Same as input
  Integrator1 : Integrator  InitialCondition=eps
  Integrator6 : Integrator
  Integrator7 : Integrator
  Product3 : Product  RndMeth=Zero
  Product4 : Product  RndMeth=Zero
  Q0 : Constant  Value=Bat_ori_cap_max_Ah
  Scope : Scope
  Switch : Switch  Criteria=u2 > Threshold  SaturateOnIntegerOverflow=off  InputSameDT=off
  To Workspace3 : ToWorkspace  VariableName=Energy_bat_consume_kWh  SaveFormat=Timeseries  SampleTime=-1
  Ws->kWh : Gain  Gain=-1/(1000*3600)
  Ws->kWh1 : Gain  Gain=-1/(1000*3600)
  SOC : Outport  InitialOutput=0
  wires:
  0 <= SOC <= 1/1 -> CD/CS mode judgement/1(SOC), SOC/1
  I_dis (A) I_chg (A)/1 -> Scope/1, Demux/1
  Demux/1 -> Icell->Ibat/1
  Demux/2 -> Icell->Ibat1/1
  Divide3/1 -> Switch/2, Product3/1, Switch/1
  Icell->Ibat/1 -> Divide3/1
  Bat dis eff/1 -> Divide3/2
  Bat chg eff/1 -> Divide4/2
  Icell->Ibat1/1 -> Divide4/1
  Divide4/1 -> Product4/2, Switch/3
  Add5/1 -> 0 <= SOC <= 1/1
  [Bat_Uoc_V] -> Product4/1, Product3/2
  Add6/1 -> To Workspace3/1
  Product3/1 -> Integrator6/1
  Integrator6/1 -> Ws->kWh/1
  Ws->kWh/1 -> Add6/1
  Product4/1 -> Integrator7/1
  Integrator7/1 -> Ws->kWh1/1
  Ws->kWh1/1 -> Add6/2
  Switch/1 -> (sec->hrs)/1
  (sec->hrs)/1 -> Integrator1/1
  Integrator1/1 -> Divide1/1
  Q0/1 -> Divide1/2
  Bat SOC0/1 -> Add5/2
  Divide1/1 -> Add5/1

== system c221127_FCEV_SLMP_SQP/Subsystem2/Electrical Model1/U0 ==
  R0 : Inport
  I : Inport  Port=2
  Demux : Demux  Outputs=2
  Switch : Switch  Criteria=u2 > Threshold  SaturateOnIntegerOverflow=off  InputSameDT=off
  U0=I*R0 : Product  RndMeth=Zero
  U0 : Outport
  wires:
  I/1 -> U0=I*R0/2, Switch/2
  R0/1 -> Demux/1
  Demux/1 -> Switch/1
  Demux/2 -> Switch/3
  Switch/1 -> U0=I*R0/1
  U0=I*R0/1 -> U0/1

== system c221127_FCEV_SLMP_SQP/Subsystem2/Electrical Model1/U1&U1 ==
  note: -V2/(C2*R2)+I/C2
  note: -V1/(C1*R1)+I/C1
  R1 : Inport
  C1 : Inport  Port=2
  R2 : Inport  Port=3
  C2 : Inport  Port=4
  I : Inport  Port=5
  Delay : Delay  DelayLength=1
  Ib/C1 : Product  Inputs=*/  RndMeth=Zero
  Ib/C2 : Product  Inputs=*/  RndMeth=Zero
  Memory1 : Memory  InitialCondition=eps  InheritSampleTime=on
  R1*C1 : Product  Inputs=**  RndMeth=Zero
  R2*C2 : Product  Inputs=**  RndMeth=Zero
  Scope : Scope  NumInputPorts=2
  Scope1 : Scope
  Sum1 : Sum
  Sum2 : Sum  Inputs=|-+
  Sum3 : Sum  Inputs=+-|
  Sum4 : Sum
  U1/(R1*C1) : Product  Inputs=*/  RndMeth=Zero
  U2/(R2*C2) : Product  Inputs=*/  RndMeth=Zero
  U1 : Outport
  U2 : Outport  Port=2
  wires:
  C1/1 -> R1*C1/1, Ib/C1/2
  I/1 -> Scope1/1, Ib/C2/1, Ib/C1/1
  R1/1 -> R1*C1/2
  R1*C1/1 -> U1/(R1*C1)/2
  U1/(R1*C1)/1 -> Sum3/2
  Ib/C1/1 -> Sum3/1
  R2/1 -> R2*C2/1
  C2/1 -> Ib/C2/2, R2*C2/2
  R2*C2/1 -> U2/(R2*C2)/2
  Ib/C2/1 -> Sum2/2
  U2/(R2*C2)/1 -> Sum2/1
  Memory1/1 -> Sum4/1, U2/(R2*C2)/1
  Sum3/1 -> Sum1/1
  Sum1/1 -> Delay/1, Scope/1, U1/1
  Sum2/1 -> Sum4/2
  Sum4/1 -> Scope/2, Memory1/1, U2/1
  Delay/1 -> U1/(R1*C1)/1, Sum1/2

== system c221127_FCEV_SLMP_SQP/Subsystem2/Thermal Model1/Calculation ==
  Cc1 : Constant  Value=62.7
  Cs : Constant  Value=4.5
  "Rc " : Constant  Value=1.94
  Rc*Cc : Product  Inputs=**  RndMeth=Zero
  Rc*Cs : Product  Inputs=**  RndMeth=Zero
  Rs : Constant  Value=3.19
  Rs*Cs : Product  Inputs=**  RndMeth=Zero
  Cc : Outport
  RcCc : Outport  Port=2
  RsCs : Outport  Port=3
  RcCs : Outport  Port=4
  wires:
  Cc1/1 -> Cc/1, Rc*Cc/1
  "Rc "/1 -> Rc*Cc/2, Rc*Cs/1
  Rc*Cc/1 -> RcCc/1
  Cs/1 -> Rs*Cs/1, Rc*Cs/2
  Rs/1 -> Rs*Cs/2
  Rc*Cs/1 -> RcCs/1
  Rs*Cs/1 -> RsCs/1

== system c221127_FCEV_SLMP_SQP/Subsystem3/FcDegCountingSubSys/Subsystem ==
  Enable : EnablePort
  Add : Sum
  Constant : Constant
  Memory : Memory
  u : Outport
  wires:
  Constant/1 -> Add/1
  Add/1 -> Memory/1
  Memory/1 -> Add/2, u/1

== system c221127_FCEV_SLMP_SQP/Subsystem3/FcDegCountingSubSys/Subsystem1 ==
  Enable : EnablePort
  Add : Sum
  Constant : Constant
  Memory : Memory
  u : Outport
  wires:
  Memory/1 -> u/1, Add/2
  Add/1 -> Memory/1
  Constant/1 -> Add/1

== system c221127_FCEV_SLMP_SQP/Subsystem4/VehModel_Pred+1/Power bus ==
  note: -
  note: +
  note: 需求制动功率
  note: 需求驱动功率
  drive power (kW) brake power (kW) req at power bus : Inport
  Constant1 : Constant  Value=DCAC_eff
  Demux2 : Demux  Outputs=2
  Divide : Product  Inputs=*/
  Divide1 : Product  Inputs=**
  Saturation : Saturate  UpperLimit=0  LowerLimit=-inf
  Saturation1 : Saturate  UpperLimit=inf  LowerLimit=0
  Switch1 : Switch  Criteria=u2 > Threshold  SaturateOnIntegerOverflow=off  InputSameDT=off
  drive power (kW)/brake power (kW) req from power sources : Outport
  wires:
  Constant1/1 -> Divide1/2, Divide/2
  Divide/1 -> Saturation1/1
  Divide1/1 -> Saturation/1
  drive power (kW) brake power (kW) req at power bus/1 -> Demux2/1
  Demux2/2 -> Divide1/1
  Saturation1/1 -> Switch1/2, Switch1/1
  Switch1/1 -> drive power (kW)/brake power (kW) req from power sources/1
  Saturation/1 -> Switch1/3
  Demux2/1 -> Divide/1

== system c221127_FCEV_SLMP_SQP/Subsystem4/VehModel_Pred+1/主减及变速器模型 ==
  drive torque (Nm) speed (rad/s) brake torque (Nm) req'd at output side of final drive : Inport
  " Effect of inertia (Nm)1" : Subsystem
  Demux4 : Demux  Outputs=3
  Effect of inertia (Nm) : Subsystem
  Gain1 : Gain  Gain=1/Veh_final_drive_ratio
  Gain2 : Gain  Gain=1/Veh_final_drive_ratio
  Gain3 : Gain  Gain=Veh_final_drive_ratio  SaturateOnIntegerOverflow=on  OutDataTypeStr=Inherit: Same as input  ParamDataTypeStr=Inherit: Same as input
  Mux4 : Mux  Inputs=3
  Sum : Sum  Inputs=+++  InputSameDT=on  SaturateOnIntegerOverflow=on  OutDataTypeStr=Inherit: Same as first input
  Sum3 : Sum  Inputs=+++  InputSameDT=on  SaturateOnIntegerOverflow=on  OutDataTypeStr=Inherit: Same as first input
  loss (Nm) : Subsystem
  loss (Nm)1 : Subsystem
  drive torque (Nm) speed (rad/s) brike torque (Nm) req'd at input side of final drive : Outport  InitialOutput=0
  wires:
  Demux4/2 -> Effect of inertia (Nm)/1(fd input speed (rad/s)), " Effect of inertia (Nm)1"/1(In1), Gain3/1
  Demux4/1 -> loss (Nm)/1("drive torque (Nm) "), Gain1/1
  Mux4/1 -> drive torque (Nm) speed (rad/s) brike torque (Nm) req'd at input side of final drive/1
  drive torque (Nm) speed (rad/s) brake torque (Nm) req'd at output side of final drive/1 -> Demux4/1
  Effect of inertia (Nm)/1(drag torque (Nm)) -> Sum/2
  loss (Nm)/1(drag torque (Nm)) -> Sum/1
  Gain1/1 -> Sum/3
  Sum/1 -> Mux4/1
  Gain3/1 -> Mux4/2
  " Effect of inertia (Nm)1"/1(Out1) -> Sum3/2
  loss (Nm)1/1(drag torque (Nm)) -> Sum3/3
  Demux4/3 -> Gain2/1, loss (Nm)1/1("drive torque (Nm) ")
  Gain2/1 -> Sum3/1
  Sum3/1 -> Mux4/3

== system c221127_FCEV_SLMP_SQP/Subsystem4/VehModel_Pred+1/整车动力学模型 ==
  需求车速 km/h : Inport
  Add1 : Sum  Inputs=++++
  Mux : Mux  Inputs=3
  compute of front axle brk from motor : Subsystem
  kmph->m/s : Gain  Gain=1/3.6
  加速阻力 : Subsystem
  坡度 : Constant  Value=0
  坡道阻力 : Subsystem
  平均车速 km/h : Scope
  整车需求驱动力 : Scope
  滚动阻力 : Subsystem
  空气阻力 : Subsystem
  需求驱动力N 目标车速m/s 需求制动力N : Outport
  wires:
  滚动阻力/1(滚动阻力 N) -> Add1/1
  坡道阻力/1(坡道阻力 N) -> Add1/2
  空气阻力/1(空气阻力 N) -> Add1/3
  加速阻力/1(加速阻力 N) -> Add1/4
  Add1/1 -> 整车需求驱动力/1, Mux/1
  Mux/1 -> 需求驱动力N 目标车速m/s 需求制动力N/1
  坡度/1 -> 坡道阻力/2(预测坡度), 滚动阻力/2(预测坡度)
  kmph->m/s/1 -> Mux/2
  需求车速 km/h/1 -> compute of front axle brk from motor/1(平均车速 km/h), kmph->m/s/1, 平均车速 km/h/1, 加速阻力/1(车速 km/h), 空气阻力/1(veh_spd km/h), 滚动阻力/1(车辆平均车速 km/h), 坡道阻力/1(车辆平均车速1)
  compute of front axle brk from motor/1(veh_front_axle_motor_brk) -> Mux/3

== system c221127_FCEV_SLMP_SQP/Subsystem4/VehModel_Pred+1/车轮模型 ==
  "tractive force, brake force and speed req'd of tire/road interface 需求驱动力N 目标车速m/s 需求制动力N" : Inport
  Add : Sum
  Add1 : Sum
  Constant : Constant  Value=0
  Demux : Demux  Outputs=3
  Gain1 : Gain  Gain=Veh_wheel_radius_m
  Gain4 : Gain  Gain=Veh_wheel_radius_m
  Interia torque : Subsystem
  Interia torque1 : Subsystem
  Mux : Mux  Inputs=3
  Switch1 : Switch  Criteria=u2 > Threshold  Threshold=15  SaturateOnIntegerOverflow=off  InputSameDT=off
  axle input speed (rad/s) : Gain  Gain=1/Veh_wheel_radius_m
  drive torque (Nm) speed (rad/s) brake torque (Nm) req'd from drivetrain into axle : Outport  InitialOutput=0
  wires:
  Demux/1 -> Gain1/1
  "tractive force, brake force and speed req'd of tire/road interface 需求驱动力N 目标车速m/s 需求制动力N"/1 -> Demux/1
  Mux/1 -> drive torque (Nm) speed (rad/s) brake torque (Nm) req'd from drivetrain into axle/1
  Gain1/1 -> Add/2
  Add/1 -> Mux/1
  Demux/2 -> axle input speed (rad/s)/1, Interia torque/1(车轮线速度 m/s), Interia torque1/1(车轮线速度 m/s)
  Interia torque/1(inertia torque (Nm)) -> Add/1
  Demux/3 -> Gain4/1
  Gain4/1 -> Add1/1
  Interia torque1/1(inertia torque (Nm)) -> Add1/2
  axle input speed (rad/s)/1 -> Switch1/2, Mux/2
  Switch1/1 -> Mux/3
  Constant/1 -> Switch1/3
  Add1/1 -> Switch1/1

== system c221127_FCEV_SLMP_SQP/Subsystem4/VehModel_Pred+1/驱动电机模型 ==
  note: nm tor per pwr w input模块*-1
      | infi和inf
  drive torque (Nm) speed (rad/s) brake torque (Nm) req'd at motor : Inport
  Brake torque_limited : Subsystem
  Constant : Constant  Value=MC_eff_dri_average
  Constant1 : Constant  Value=MC_eff_brk_average
  Demux2 : Demux  Outputs=3
  Divide : Product  Inputs=/*
  Divide1 : Product  Inputs=**
  Drive torque_limited : Subsystem
  Inertia torque : Subsystem
  Inertia torque1 : Subsystem
  Motor brake output power (kW) : Lookup2D  RowIndex=MC_ori_spd_rpm*MC_spd_scale  ColumnIndex=MC_ori_trq_brk_Nm*MC_trq_scale  Table=MC_ori_power_brk_req_kW*MC_spd_scale*MC_trq_scale
  Motor drive output power (kW) : Lookup2D  RowIndex=MC_ori_spd_rpm*MC_spd_scale  ColumnIndex=MC_ori_trq_dri_Nm*MC_trq_scale  Table=MC_ori_power_dri_req_kW*MC_spd_scale*MC_trq_scale
  Mux : Mux  Inputs=2
  Saturation : Saturate  UpperLimit=MC_spd_max_rpm  LowerLimit=MC_spd_min_rpm
  Saturation1 : Saturate  UpperLimit=MC_power_max_kW  LowerLimit=0  LinearizeAsGain=off
  Saturation2 : Saturate  UpperLimit=0  LowerLimit=-MC_power_max_kW
  Sum2 : Sum  InputSameDT=on  SaturateOnIntegerOverflow=on  OutDataTypeStr=Inherit: Same as first input
  Sum3 : Sum  InputSameDT=on  SaturateOnIntegerOverflow=on  OutDataTypeStr=Inherit: Same as first input
  rad/s->rpm1 : Gain  Gain=60/(2*pi)
  drive power (kW) brake power (kW) req'd motor input power (电功率) : Outport  InitialOutput=0
  wires:
  drive torque (Nm) speed (rad/s) brake torque (Nm) req'd at motor/1 -> Demux2/1
  rad/s->rpm1/1 -> Saturation/1
  Demux2/2 -> rad/s->rpm1/1
  Demux2/1 -> Sum2/2
  Inertia torque/1(Out1) -> Sum2/1
  Sum2/1 -> Drive torque_limited/1(tor_req nm)
  Drive torque_limited/1(limted mc torque nm) -> Motor drive output power (kW)/2
  Motor drive output power (kW)/1 -> Saturation1/1
  Constant/1 -> Divide/1
  Divide/1 -> Mux/1
  Mux/1 -> drive power (kW) brake power (kW) req'd motor input power (电功率)/1
  Demux2/3 -> Sum3/1
  Inertia torque1/1(Out1) -> Sum3/2
  Sum3/1 -> Brake torque_limited/1(tor_req nm)
  Motor brake output power (kW)/1 -> Saturation2/1
  Saturation2/1 -> Divide1/1
  Constant1/1 -> Divide1/2
  Divide1/1 -> Mux/2
  Saturation1/1 -> Divide/2
  Brake torque_limited/1(limted mc torque nm) -> Motor brake output power (kW)/2
  Saturation/1 -> Inertia torque1/1(motor spd rpm), Brake torque_limited/2(mc spd rpm), Motor brake output power (kW)/1, Motor drive output power (kW)/1, Drive torque_limited/2(mc spd rpm), Inertia torque/1(motor spd rpm)

== system c221127_FCEV_SLMP_SQP/Subsystem4/VehModel_Pred+2/Power bus ==
  note: -
  note: +
  note: 需求制动功率
  note: 需求驱动功率
  drive power (kW) brake power (kW) req at power bus : Inport
  Constant1 : Constant  Value=DCAC_eff
  Demux2 : Demux  Outputs=2
  Divide : Product  Inputs=*/
  Divide1 : Product  Inputs=**
  Saturation : Saturate  UpperLimit=0  LowerLimit=-inf
  Saturation1 : Saturate  UpperLimit=inf  LowerLimit=0
  Switch1 : Switch  Criteria=u2 > Threshold  SaturateOnIntegerOverflow=off  InputSameDT=off
  drive power (kW)/brake power (kW) req from power sources : Outport
  wires:
  Constant1/1 -> Divide1/2, Divide/2
  Divide/1 -> Saturation1/1
  Divide1/1 -> Saturation/1
  drive power (kW) brake power (kW) req at power bus/1 -> Demux2/1
  Demux2/2 -> Divide1/1
  Saturation1/1 -> Switch1/2, Switch1/1
  Switch1/1 -> drive power (kW)/brake power (kW) req from power sources/1
  Saturation/1 -> Switch1/3
  Demux2/1 -> Divide/1

== system c221127_FCEV_SLMP_SQP/Subsystem4/VehModel_Pred+2/主减及变速器模型 ==
  drive torque (Nm) speed (rad/s) brake torque (Nm) req'd at output side of final drive : Inport
  " Effect of inertia (Nm)1" : Subsystem
  Demux4 : Demux  Outputs=3
  Effect of inertia (Nm) : Subsystem
  Gain1 : Gain  Gain=1/Veh_final_drive_ratio
  Gain2 : Gain  Gain=1/Veh_final_drive_ratio
  Gain3 : Gain  Gain=Veh_final_drive_ratio  SaturateOnIntegerOverflow=on  OutDataTypeStr=Inherit: Same as input  ParamDataTypeStr=Inherit: Same as input
  Mux4 : Mux  Inputs=3
  Sum : Sum  Inputs=+++  InputSameDT=on  SaturateOnIntegerOverflow=on  OutDataTypeStr=Inherit: Same as first input
  Sum3 : Sum  Inputs=+++  InputSameDT=on  SaturateOnIntegerOverflow=on  OutDataTypeStr=Inherit: Same as first input
  loss (Nm) : Subsystem
  loss (Nm)1 : Subsystem
  drive torque (Nm) speed (rad/s) brike torque (Nm) req'd at input side of final drive : Outport  InitialOutput=0
  wires:
  Demux4/2 -> Effect of inertia (Nm)/1(fd input speed (rad/s)), " Effect of inertia (Nm)1"/1(In1), Gain3/1
  Demux4/1 -> loss (Nm)/1("drive torque (Nm) "), Gain1/1
  Mux4/1 -> drive torque (Nm) speed (rad/s) brike torque (Nm) req'd at input side of final drive/1
  drive torque (Nm) speed (rad/s) brake torque (Nm) req'd at output side of final drive/1 -> Demux4/1
  Effect of inertia (Nm)/1(drag torque (Nm)) -> Sum/2
  loss (Nm)/1(drag torque (Nm)) -> Sum/1
  Gain1/1 -> Sum/3
  Sum/1 -> Mux4/1
  Gain3/1 -> Mux4/2
  " Effect of inertia (Nm)1"/1(Out1) -> Sum3/2
  loss (Nm)1/1(drag torque (Nm)) -> Sum3/3
  Demux4/3 -> Gain2/1, loss (Nm)1/1("drive torque (Nm) ")
  Gain2/1 -> Sum3/1
  Sum3/1 -> Mux4/3

== system c221127_FCEV_SLMP_SQP/Subsystem4/VehModel_Pred+2/整车动力学模型 ==
  需求车速 km/h : Inport
  Temp : Inport  Port=2
  Add1 : Sum  Inputs=++++
  Mux : Mux  Inputs=3
  compute of front axle brk from motor : Subsystem
  kmph->m/s : Gain  Gain=1/3.6
  加速阻力 : Subsystem
  坡度 : Constant  Value=0
  坡道阻力 : Subsystem
  平均车速 km/h : Scope
  整车需求驱动力 : Scope
  滚动阻力 : Subsystem
  空气阻力 : Subsystem
  需求驱动力N 目标车速m/s 需求制动力N : Outport
  wires:
  滚动阻力/1(滚动阻力 N) -> Add1/1
  坡道阻力/1(坡道阻力 N) -> Add1/2
  空气阻力/1(空气阻力 N) -> Add1/3
  需求车速 km/h/1 -> compute of front axle brk from motor/1(平均车速 km/h), kmph->m/s/1, 平均车速 km/h/1, 加速阻力/1(车速 km/h), 空气阻力/1(veh_spd km/h), 滚动阻力/1(车辆平均车速 km/h), 坡道阻力/1(车辆平均车速1)
  Add1/1 -> 整车需求驱动力/1, Mux/1
  Mux/1 -> 需求驱动力N 目标车速m/s 需求制动力N/1
  坡度/1 -> 坡道阻力/2(预测坡度), 滚动阻力/2(预测坡度)
  kmph->m/s/1 -> Mux/2
  compute of front axle brk from motor/1(veh_front_axle_motor_brk) -> Mux/3
  加速阻力/1(加速阻力 N) -> Add1/4
  Temp/1 -> 加速阻力/2(车速 km/h1)

== system c221127_FCEV_SLMP_SQP/Subsystem4/VehModel_Pred+2/车轮模型 ==
  "tractive force, brake force and speed req'd of tire/road interface 需求驱动力N 目标车速m/s 需求制动力N" : Inport
  Add : Sum
  Add1 : Sum
  Constant : Constant  Value=0
  Demux : Demux  Outputs=3
  Gain1 : Gain  Gain=Veh_wheel_radius_m
  Gain4 : Gain  Gain=Veh_wheel_radius_m
  Interia torque : Subsystem
  Interia torque1 : Subsystem
  Mux : Mux  Inputs=3
  Switch1 : Switch  Criteria=u2 > Threshold  Threshold=15  SaturateOnIntegerOverflow=off  InputSameDT=off
  axle input speed (rad/s) : Gain  Gain=1/Veh_wheel_radius_m
  drive torque (Nm) speed (rad/s) brake torque (Nm) req'd from drivetrain into axle : Outport  InitialOutput=0
  wires:
  Demux/1 -> Gain1/1
  "tractive force, brake force and speed req'd of tire/road interface 需求驱动力N 目标车速m/s 需求制动力N"/1 -> Demux/1
  Mux/1 -> drive torque (Nm) speed (rad/s) brake torque (Nm) req'd from drivetrain into axle/1
  Gain1/1 -> Add/2
  Add/1 -> Mux/1
  Demux/2 -> axle input speed (rad/s)/1, Interia torque/1(车轮线速度 m/s), Interia torque1/1(车轮线速度 m/s)
  Interia torque/1(inertia torque (Nm)) -> Add/1
  Demux/3 -> Gain4/1
  Gain4/1 -> Add1/1
  Interia torque1/1(inertia torque (Nm)) -> Add1/2
  axle input speed (rad/s)/1 -> Switch1/2, Mux/2
  Switch1/1 -> Mux/3
  Constant/1 -> Switch1/3
  Add1/1 -> Switch1/1
